simulink model "symulacja4"  (R2025b)
settings: Solver=VariableStepAuto  StartTime=0.0  StopTime=1000  MaxStep=0.1  RelTol=1e-3
values from neighbouring files (symbols this model uses):
  k = delta_x / delta_u    [skrypt3.m]    (also in skrypt4.m)
  kp = 0.9*T/(k*t_0)    [skrypt4.m]
  przy_sp = 5    [skrypt4.m]
  step_time = 400    [skrypt2.m]    (also in skrypt3.m = 10; skrypt4.m = 100)
  T = 247    [skrypt3.m]    (also in skrypt4.m)
  t_0 = 13    [skrypt3.m]    (also in skrypt4.m)
  ti = 3.33*t_0    (= 43.29)    [skrypt4.m]
  Tkz0 = tab_tk(i)    [skrypt2.m]    (also in skrypt3.m = 30; skrypt4.m = 30)
  Tw2c = ((A + Ks1 + K0)*Ks2*Tzew0 + K0*(A*Tkz0 + Ks1*Tzew0)) / ((A + Ks1 + K0)*(K0 + Ks2) - K0^2)    [skrypt2.m]    (also in skrypt3.m = 15; skrypt4.m = 15)
settings Model: Creator=mikol  LastModifiedBy=mikol

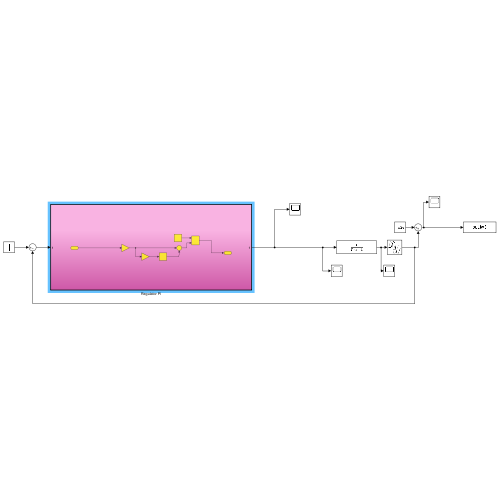
[thumbnail: Simulink's stored preview of the top-level diagram]
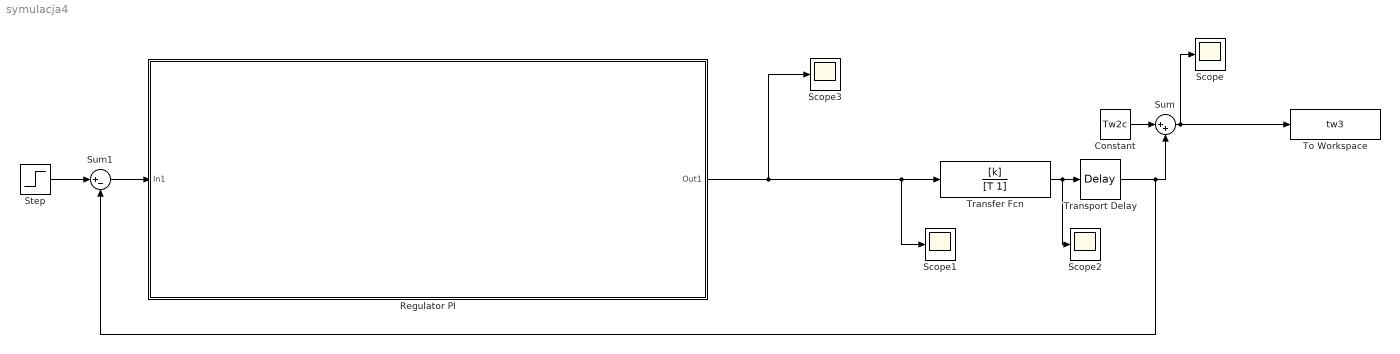
== system symulacja4 ==
  Constant : Constant  Value=Tw2c
  Regulator PI : Subsystem  TreatAsAtomicUnit=on
  Scope{,1..3} (4 alike) : Scope
      Scope settings: ActiveDisplayYMinimum=14.238082536293582  ActiveDisplayYMaximum=33.083673858522125
      Scope1 settings: ActiveDisplayYMinimum=-1  ActiveDisplayYMaximum=1
      Scope2 settings: ActiveDisplayYMinimum=-1  ActiveDisplayYMaximum=1  DataLoggingVariableName=ScopeData2
      Scope3 settings: ActiveDisplayYMinimum=-65.43540098032814  ActiveDisplayYMaximum=77.161359782530454  DataLoggingVariableName=ScopeData3
  Step : Step  Time=step_time  After=przy_sp  SampleTime=0
  Sum : Sum  Inputs=|++
  Sum1 : Sum  Inputs=|+-
  To Workspace : ToWorkspace  VariableName=tw3  SampleTime=-1
  Transfer Fcn : TransferFcn  Numerator=[k]  Denominator=[T 1]
  Transport Delay : TransportDelay  DelayTime=t_0
  wires:
  Transport Delay/1 -> Sum1/2, Sum/2
  Transfer Fcn/1 -> Scope2/1, Transport Delay/1
  Regulator PI/1(Out1) -> Scope3/1, Transfer Fcn/1, Scope1/1
  Sum/1 -> Scope/1, To Workspace/1
  Step/1 -> Sum1/1
  Sum1/1 -> Regulator PI/1(In1)
  Constant/1 -> Sum/1

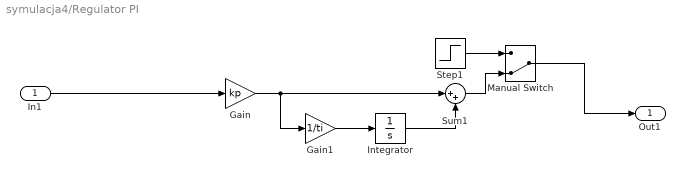
== system symulacja4/Regulator PI ==
  In1 : Inport
  Gain : Gain  Gain=kp
  Gain1 : Gain  Gain=1/ti
  Integrator : Integrator  InitialCondition=Tkz0
  Manual Switch : ManualSwitch  CurrentSetting=0
  Step1 : Step  Time=step_time  After=przy_sp  SampleTime=0
  Sum1 : Sum  Inputs=|++
  Out1 : Outport
  wires:
  Manual Switch/1 -> Out1/1
  Step1/1 -> Manual Switch/1
  Gain/1 -> Sum1/1, Gain1/1
  Gain1/1 -> Integrator/1
  Integrator/1 -> Sum1/2
  Sum1/1 -> Manual Switch/2
  In1/1 -> Gain/1
